simulink model "my_pc_surveil_tcpip"  (Simulink 7.1)
settings: Solver=FixedStepDiscrete  SolverMode=SingleTasking  StartTime=0.0  StopTime=inf  RelTol=1e-3
libraries: etargetslib x2, vipsnks x2, instrumentlib x2, simulink x1, viptextngfix x1, dspsigops x1, dspobslib x1, dspsrcs4 x1
settings Model: Creator=don  LastModifiedBy=karin  ExtModeAutoUpdateStatusClock=off
settings DataIOCC: SaveOutput=off  SaveTime=off  SignalLoggingName=sigsOut
settings DebuggingCC: CheckExecutionContextPreStartOutputMsg=on  CheckExecutionContextRuntimeOutputMsg=on  SignalResolutionControl=TryResolveAllWithWarning  SolverPrmCheckMsg=none  MultiTaskDSMMsg=warning  MultiTaskCondExecSysMsg=none  ParameterPrecisionLossMsg=none  StrictBusMsg=None
settings HardwareCC: TargetUnknown=on
settings RTWCC: IncludeERTFirstTime=on
settings GRTTargetCC: TargetFcnLib=ansi_tfl_tmw_new.mat

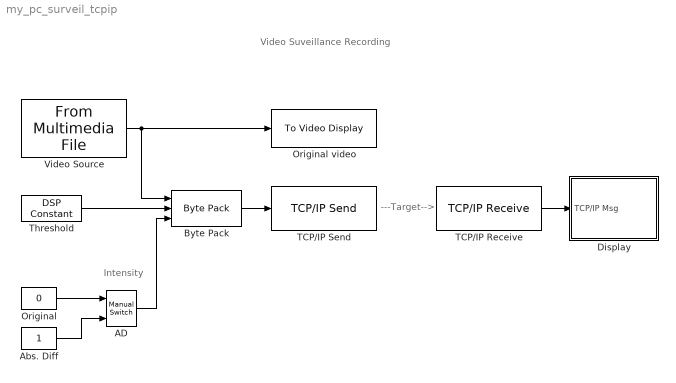
== system my_pc_surveil_tcpip ==
  note: Video Suveillance Recording
  note: ---Target-->
  note: Intensity
  AD : simulink/Signal Routing/Manual Switch  SystemSampleTime=-1  sw=1  action=0  varsize=off
  Abs. Diff : Constant  OutDataTypeMode=boolean  OutDataType=sfix(16)  OutScaling=2^0  OutDataTypeStr=boolean
  Byte Pack : etargetslib/Byte Pack  datatypes={'uint8','int32','boolean'}  byteAlign=1
  Display : Subsystem
  Original : Constant  Value=0  OutDataTypeMode=boolean  OutDataType=sfix(16)  OutScaling=2^0  OutDataTypeStr=boolean
  Original video : vipsnks/To Video Display  DialogController=vipDDGCreate  DialogControllerArgs=DataTag2  inputType=Obsolete  imagePorts=One multidimensional signal  OutputDevice=On-screen video monitor  fullScreen=off  videoWindowX=347  videoWindowY=358  saveWindowSize=off  videoWindowWidth=168  videoWindowHeight=147  dataOrg=Column-major
  TCP/IP Receive : instrumentlib/TCP//IP Receive  Priority=10  DialogController=instrumentcreatedialog  DialogControllerArgs=DataTag3  Host=132.66.49.63  Port=49000  DataSize="[1  19212]"  EnableBlockingMode=on  Timeout=3  SampleTime=1/30  DataType=uint8  ByteOrder=BigEndian
  TCP/IP Send : instrumentlib/TCP//IP Send  Priority=5  DialogController=instrumentcreatedialog  DialogControllerArgs=DataTag4  Host=132.66.49.63  Port=49000  EnableBlockingMode=on  Timeout=3  ByteOrder=BigEndian
  Threshold : dspobslib/DSP Constant  SystemSampleTime=-1  Value=1e5  SampleMode=Discrete  discreteOutput=Sample-based  continuousOutput=Sample-based  sampTime=Inf  framePeriod=Inf  dataType=int32  isSigned=on  wordLen=16  udDataType=sfix(16)  fracBitsMode=Best precision  numFracBits=15  InterpretAs1D=off  Ts=Inf  FramebasedOutput=off
      settings: additionalParams=on
  Video Source : dspsrcs4/From Multimedia File  Priority=1  DialogController=dspDDGCreate  DialogControllerArgs=DataTag5  inputFilename=vipmen.avi  loop=on  numPlays=inf  outputStreams=Video only  videoDataType=uint8  audioDataType=int16  inheritSampleTime=on  userDefinedSampleTime=1/30  noAudioOutput=off  isIntensityVideo=on  colorVideoFormat=Separate color signals  outputEOF=off  dataOrg=Column-major
  wires:
  Video Source/1 -> Original video/1, Byte Pack/1
  Threshold/1 -> Byte Pack/2
  Byte Pack/1 -> TCP/IP Send/1
  TCP/IP Receive/1 -> Display/1(TCP/IP Msg)
  Original/1 -> AD/1
  Abs. Diff/1 -> AD/2
  AD/1 -> Byte Pack/3

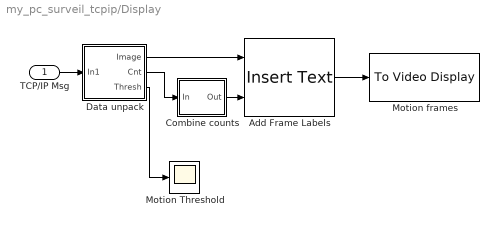
== system my_pc_surveil_tcpip/Display ==
  TCP/IP Msg : Inport  OutDataType=sfix(16)  OutScaling=2^0
  Add Frame Labels : viptextngfix/Insert Text  DialogController=vipDDGCreate  DialogControllerArgs=DataTag0  inputType=Obsolete  theText=['Source frame: %d' sprintf('\n') 'Captured frame: %d']  fontFace=LucidaSansRegular  dummyVar1=0  blockFontSize=12  antiAliased=on  getTextLocFrom=Specify via dialog  textLoc=[93 2]  getTextColorFrom=Specify via dialog  textColor=255  getTextIntensityFrom=Specify via dialog  textIntensity=255  getTextOpacityFrom=Specify via dialog  textOpacity=1.0  dummyVar2=0  dummyVar3=0  dummyVar4=0  imagePorts=One multidimensional signal  isInputTransposed=off
  Combine counts : Subsystem
  Data unpack : Subsystem
  Motion Threshold : Scope
      settings: TimeRange=10  YMin=0  YMax=200000
  Motion frames : vipsnks/To Video Display  DialogController=vipDDGCreate  DialogControllerArgs=DataTag1  inputType=Intensity  imagePorts=One multidimensional signal  OutputDevice=On-screen video monitor  fullScreen=off  videoWindowX=526  videoWindowY=358  saveWindowSize=off  videoWindowWidth=168  videoWindowHeight=147  dataOrg=Column-major
  wires:
  Add Frame Labels/1 -> Motion frames/1
  Data unpack/1(Image) -> Add Frame Labels/1
  Combine counts/1(Out) -> Add Frame Labels/2
  Data unpack/2(Cnt) -> Combine counts/1(In)
  Data unpack/3(Thresh) -> Motion Threshold/1
  TCP/IP Msg/1 -> Data unpack/1(In1)

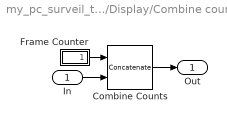
== system my_pc_surveil_tcpip/Display/Combine counts ==
  In : Inport  OutDataType=sfix(16)  OutScaling=2^0
  Combine Counts : Concatenate  Mode=Multidimensional array  ConcatenateDimension=2
  Frame Counter : Subsystem
  Out : Outport  OutDataType=sfix(16)  OutScaling=2^0
  wires:
  Frame Counter/1(" Cnt") -> Combine Counts/1
  Combine Counts/1 -> Out/1
  In/1 -> Combine Counts/2

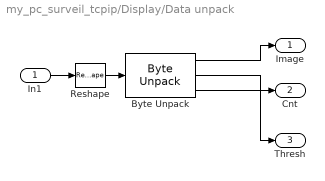
== system my_pc_surveil_tcpip/Display/Data unpack ==
  In1 : Inport  OutDataType=sfix(16)  OutScaling=2^0
  Byte Unpack : etargetslib/Byte Unpack  dimensions={[120, 160],[1],[2,1]}  datatypes={'uint8','int32','int32'}  byteAlign=1
  Reshape : Reshape
  Image : Outport  OutDataType=sfix(16)  OutScaling=2^0
  Cnt : Outport  Port=2  OutDataType=sfix(16)  OutScaling=2^0
  Thresh : Outport  Port=3  OutDataType=sfix(16)  OutScaling=2^0
  wires:
  Reshape/1 -> Byte Unpack/1
  Byte Unpack/1 -> Image/1
  Byte Unpack/2 -> Cnt/1
  In1/1 -> Reshape/1
  Byte Unpack/3 -> Thresh/1

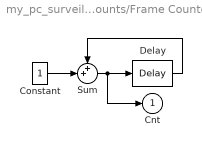
== system my_pc_surveil_tcpip/Display/Combine counts/Frame Counter ==
  Constant : Constant  OutDataTypeMode=int32  OutDataType=sfix(16)  OutScaling=2^0  OutDataTypeStr=int32
  Delay : dspsigops/Delay  dly_unit=Samples  delay=1  ic_detail=off  dif_ic_for_ch=off  dif_ic_for_dly=off  ic=0  reset_popup=None
  Sum : Sum  Inputs=++|  OutDataType=sfix(16)  OutScaling=2^0  OutDataTypeStr=Inherit: Same as first input
  " Cnt" : Outport  OutDataType=sfix(16)  OutScaling=2^0
  wires:
  Constant/1 -> Sum/2
  Sum/1 -> Delay/1, " Cnt"/1
  Delay/1 -> Sum/1
